simulink model "Lab_4_sim"  (R2020a)
settings: Solver=VariableStepAuto  StartTime=0.0  StopTime=100  RelTol=1e-3
values from neighbouring files (symbols this model uses):
  L = KR_d.Numerator{1, 1}    [Lab_4.m]
  M = Kr_d.Denominator{1, 1}    [Lab_4.m]
  TS = 0.1    [Lab_4.m]
libraries: simulink x1
settings Model: Creator=Piotr  LastModifiedBy=Piotr

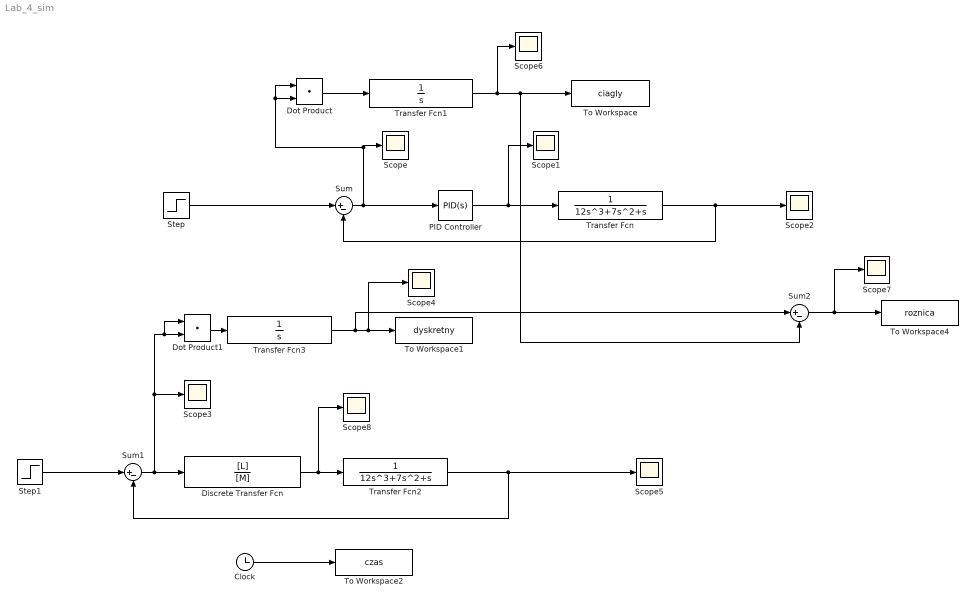
== system Lab_4_sim ==
  Clock : Clock
      settings: Decimation=100
  Discrete Transfer Fcn : DiscreteTransferFcn  Numerator=[L]  Denominator=[M]  SampleTime=TS
  Dot Product : DotProduct  InputSameDT=on  OutDataTypeStr=Inherit: Inherit via internal rule
  Dot Product1 : DotProduct  InputSameDT=on  OutDataTypeStr=Inherit: Inherit via internal rule
  PID Controller : simulink/Continuous/PID Controller  Controller=PID  Form=Parallel  TimeDomain=Continuous-time  UseExternalTs=off  SampleTime=-1  IntegratorMethod=Forward Euler  FilterMethod=Forward Euler  ControllerParametersSource=internal  P=0.289702409757857  I=0.00677268499129384  D=2.00668283519911  UseFilter=on  N=35.184355111403  TunerSelectOption=Transfer Function Based (PID Tuner App)  InitialConditionSource=internal  InitialConditionForIntegrator=0  InitialConditionForFilter=0  DifferentiatorICPrevScaledInput=0  ExternalReset=none  TrackingMode=off  Kt=1  LimitOutput=off  UpperSaturationLimit=inf  LowerSaturationLimit=-inf  LinearizeAsGain=on  AntiWindupMode=none  Kb=1  POutMin=[]  POutMax=[]  IOutMin=[]  IOutMax=[]  DOutMin=[]  DOutMax=[]  NOutMin=[]  NOutMax=[]  SumOutMin=[]  SumOutMax=[]  SaturationOutMin=[]  SaturationOutMax=[]  PParamMin=[]  PParamMax=[]  IParamMin=[]  IParamMax=[]  DParamMin=[]  DParamMax=[]  NParamMin=[]  NParamMax=[]  KbParamMin=[]  KbParamMax=[]  KtParamMin=[]  KtParamMax=[]  KbOutMin=[]  KbOutMax=[]  KtOutMin=[]  KtOutMax=[]  IntegratorOutMin=[]  IntegratorOutMax=[]  FilterOutMin=[]  FilterOutMax=[]  SumI1OutMin=[]  SumI1OutMax=[]  SumI2OutMin=[]  SumI2OutMax=[]  SumI3OutMin=[]  SumI3OutMax=[]  SumI4OutMin=[]  SumI4OutMax=[]  SumDOutMin=[]  SumDOutMax=[]  DifferentiatorOutMin=[]  DifferentiatorOutMax=[]  FilterDiffOutCoefMin=[]  FilterDiffOutCoefMax=[]  ReciprocalOutMin=[]  ReciprocalOutMax=[]  SumDenOutMin=[]  SumDenOutMax=[]  SumNumOutMin=[]  SumNumOutMax=[]  DivideOutMin=[]  DivideOutMax=[]  UdiffTsProdOutMin=[]  UdiffTsProdOutMax=[]  NTsProdOutMin=[]  NTsProdOutMax=[]  UintegralTsProdOutMin=[]  UintegralTsProdOutMax=[]  UngainTsProdOutMin=[]  UngainTsProdOutMax=[]  IntegratorContinuousStateAttributes=''  IntegratorStateMustResolveToSignalObject=off  IntegratorRTWStateStorageClass=Auto  FilterContinuousStateAttributes=''  FilterStateMustResolveToSignalObject=off  FilterRTWStateStorageClass=Auto  ParallelPVariant=InternalParameters  IdealPVariant=Disabled  IVariant=InternalParameters  DVariant=InternalParameters  IntegratorVariant=Continuous  SatVariant=Disabled  AWVariant=Passthrough  PCopyVariant=Disabled  TRVariant=Disabled  FdbkBlocksVariant=Forward  IdealPFdbkVariant=Disabled  SatFdbkVariant=Disabled  DerivativeFilterVariant=ContFilter  NVariant=InternalParameters  NCopyVariant=Disabled  FilterICVariant=InternalICsFilter  IntegratorICVariant=InternalICs  ExternalResetVariant=Disabled  TRSumVariant=Passthrough  SumFdbkVariant=Disabled  SumVariant=Sum_PID  TsampFilterVariant=InternalTs  TsampNgainVariant=Passthrough  TsampIntegralVariant=Passthrough
  Scope{,1..8} (9 alike) : Scope
  Step : Step  SampleTime=0
  Step1 : Step  SampleTime=0
  Sum : Sum  Inputs=|+-
  Sum1 : Sum  Inputs=|+-
  Sum2 : Sum  Inputs=|+-
  To Workspace : ToWorkspace  VariableName=ciagly  SampleTime=-1
  To Workspace1 : ToWorkspace  VariableName=dyskretny  SampleTime=-1
  To Workspace2 : ToWorkspace  VariableName=czas  SampleTime=-1
  To Workspace4 : ToWorkspace  VariableName=roznica  SampleTime=-1
  Transfer Fcn : TransferFcn  Denominator=[12 7 1 0]
  Transfer Fcn1 : TransferFcn  Denominator=[1 0]
  Transfer Fcn2 : TransferFcn  Denominator=[12 7 1 0]
  Transfer Fcn3 : TransferFcn  Denominator=[1 0]
  wires:
  Step/1 -> Sum/1
  Sum/1 -> Dot Product/1, Dot Product/2, Scope/1, PID Controller/1
  Discrete Transfer Fcn/1 -> Scope8/1, Transfer Fcn2/1
  PID Controller/1 -> Scope1/1, Transfer Fcn/1
  Transfer Fcn/1 -> Scope2/1, Sum/2
  Clock/1 -> To Workspace2/1
  Dot Product/1 -> Transfer Fcn1/1
  Transfer Fcn1/1 -> Scope6/1, Sum2/2, To Workspace/1
  Step1/1 -> Sum1/1
  Transfer Fcn2/1 -> Scope5/1, Sum1/2
  Sum1/1 -> Discrete Transfer Fcn/1, Dot Product1/1, Dot Product1/2, Scope3/1
  Dot Product1/1 -> Transfer Fcn3/1
  Transfer Fcn3/1 -> Sum2/1, Scope4/1, To Workspace1/1
  Sum2/1 -> Scope7/1, To Workspace4/1
